simulink model "Hybrid_PV_Wind_System"  (R2018a)
settings: Solver=ode3  StartTime=0.0  StopTime=80  FixedStep=1e-4  RelTol=1e-3  EnableMultiTasking=on
InitFcn:
  | clear all ;
  | clc;
  | 
  | %%Wind System%%
  | 
  | %wind speed
  | Z_data=10;
  | Z_hub=85;
  | Z_0=0.03;
  | 
  | %Turbine
  | R_=45;
  | G=100;
  | lambda_opt=7.07;
  | Rho=1.225;
  | J=254;
  | f=0.01;
  | 
  | %RL filter;
  | 
  | fs=10000;
  | fe=50;
  | Ws=2*pi*fe;
  | Pres=3e6;
  | L=0.75e-3;
  | R=0.075;
  | c=38e-3;
  | 
  | %Commande CCR;
  | 
  | Id_=0;
  | Vdc_=1200;
  | %Vq_=0;
  | tr=0.001;
  | kp=3*L/tr;
  | ki=3*R/tr;
  | 
  | %CCM Commande;
  | 
  | p=2;
  | Tr=0.02;
  | Lfs=121e-6;
  | Lfr=57.3e-6;
  | Lm=12.12e-3;
  | m=1;
  | Ls=Lfs+Lm;
  | Lr=Lfr+m*Lm;
  | sigma=1-(m*Lm)^2/(Ls*Lr);
  | Rr=3.82e-3;
  | Rs=2.97e-3;
  | kpr=3*sigma*Lr/Tr;
  | kir=3*Rr/Tr;
  | Qs_ref=0;
  | 
  | %%PV SYSTEM%%
  | 
  | % T_cellule;
  | NOCT=45;
  | 
  | %PV module;
  | ... (+42 lines)
undefined symbols (not defined in the file): sigbuilder_block
libraries: powerlib_meascontrol x20, simulink x10
(part 2 of 2)

== system Hybrid_PV_Wind_System/August/Temperature8 ==
  Demux : Demux  Tag=STV Demux  Outputs=1
      settings: DisplayOption=none
  FromWs : FromWorkspace  Tag=STV FromWs  VariableName=tuvar
      SigBuilderData=|
      | common.afterFinalStr = 'Extrapolate'
      | common.sampleTime = 0
      | dataSet.timeRange = [0 745]
      | dataSet.name = 'Group 1'
      | sbobj.Groups.Name = 'Group 1'
      | sbobj.Groups.Signals.Name = 'Signal 1'
      | sbobj.Groups.Signals.XData = [0 1 2 3 4 5 6 7 8 9 10 11 ... (745 elements, 1x745)]
      | sbobj.Groups.Signals.YData = [35.7 34 32.3 31.4 30.5 29.9 29.9 31.6 33.8 36 38.1 40 ... (745 elements, 1x745)]
      | sbobj.Groups.TimeRange = [0 745]
  Signal 1 : Outport  Tag=STV Outport
  wires:
  FromWs/1 -> Demux/1
  Demux/1 -> Signal 1/1

== system Hybrid_PV_Wind_System/August/Three Phase DC AC inverter ==
  Vdc : Inport
  pwma : Inport  Port=2
  pwmb : Inport  Port=3
  pwmc : Inport  Port=4
  Fcn : Fcn  Expr=u(1)/6*(2*u(2)-u(3)-u(4))
  Fcn1 : Fcn  Expr=u(1)/6*(-u(2)+2*u(3)-u(4))
  Fcn2 : Fcn  Expr=u(1)/6*(-u(2)-u(3)+2*u(4))
  Mux : Mux
  Via : Outport
  Vib : Outport  Port=2
  Vic : Outport  Port=3
  wires:
  Vdc/1 -> Mux/1
  Mux/1 -> Fcn2/1, Fcn1/1, Fcn/1
  Fcn2/1 -> Vic/1
  Fcn1/1 -> Vib/1
  Fcn/1 -> Via/1
  pwma/1 -> Mux/2
  pwmb/1 -> Mux/3
  pwmc/1 -> Mux/4

== system Hybrid_PV_Wind_System/August/Turbine ==
  note: T_aero
  note: omega_t
  note: omega
  note: lambda
  note: Cp
  S : Inport
  B : Inport  Port=2
  1/lambda_i : Fcn  Expr=1/(u(1)+0.08*u(2))-0.035/(2^3+1)
  Cp(lambda,B) : Fcn  Expr=0.5176*(116*u(2)-0.4*u(3)-5)*exp(-21*u(2))+0.0068*u(1)
  Gain : Gain  Gain=R_/G
  Gain1 : Gain  Gain=1/G
  Gain2 : Gain  Gain=1/G
  Gain3 : Gain  Gain=lambda_opt*G/R_
  Gain5 : Gain  Gain=-1
  Mux : Mux  Inputs=2
  Mux1 : Mux  Inputs=3
  Mux2 : Mux  Inputs=3
  Mux3 : Mux  Inputs=2
  Product : Product  Inputs=*/
  Saturation : Saturate  UpperLimit=200  LowerLimit=0
  Saturation1 : Saturate  UpperLimit=0  LowerLimit=-3e6
  Saturation2 : Saturate  UpperLimit=200  LowerLimit=0
  Scope{1..5} (5 alike) : Scope
  Subsystem : Subsystem
  Subsystem1 : Subsystem
  Subsystem8 : Subsystem
  Taero(S,cp) : Fcn  Expr=0.5*u(1)*Rho*pi*(R_^2)*(u(2)^3)/u(3)
  omega : Outport
  Ps* : Outport  Port=2
  wires:
  Subsystem8/1(Ps*) -> Saturation1/1
  1/lambda_i/1 -> Mux1/2
  B/1 -> Mux1/3, Mux3/2
  Product/1 -> Mux3/1, Mux1/1
  S/1 -> Gain3/1, Mux2/2, Product/2
  Cp(lambda,B)/1 -> Mux2/1
  Gain/1 -> Product/1
  Gain2/1 -> Mux2/3
  Mux1/1 -> Cp(lambda,B)/1
  Mux2/1 -> Taero(S,cp)/1
  Taero(S,cp)/1 -> Gain1/1
  Mux/1 -> Scope1/1
  Mux3/1 -> 1/lambda_i/1
  Gain5/1 -> Subsystem8/1(Tem*), Scope3/1
  Subsystem1/1(Tem) -> Subsystem/2(Tem), Gain5/1
  Gain1/1 -> Scope5/1, Subsystem1/1(Tt), Subsystem/1(Tt)
  Gain3/1 -> Saturation/1, Mux/1
  Saturation/1 -> Subsystem1/2(omega_ref)
  Saturation1/1 -> Scope4/1, Ps*/1
  Subsystem/1(omega) -> Saturation2/1
  Saturation2/1 -> omega/1, Scope2/1, Gain/1, Gain2/1, Mux/2, Subsystem1/3(omega), Subsystem8/2(omega)

== system Hybrid_PV_Wind_System/August/Wind speed8 ==
  Demux : Demux  Tag=STV Demux  Outputs=1
      settings: DisplayOption=none
  FromWs : FromWorkspace  Tag=STV FromWs  VariableName=tuvar
      SigBuilderData=|
      | common.afterFinalStr = 'Extrapolate'
      | common.sampleTime = 0
      | dataSet.timeRange = [0 750]
      | dataSet.name = 'Group 1'
      | sbobj.Groups.Name = 'Group 1'
      | sbobj.Groups.Signals.Name = 'Signal 2'
      | sbobj.Groups.Signals.XData = [0 1 2 3 4 5 6 7 8 9 10 11 ... (744 elements, 1x744)]
      | sbobj.Groups.Signals.YData = [7.2 6.9 7.1 7.1 4.6 5.7 4.8 5.2 4.4 6.2 7.7 8.7 ... (744 elements, 1x744)]
      | sbobj.Groups.TimeRange = [0 750]
  Signal 2 : Outport  Tag=STV Outport
  wires:
  Demux/1 -> Signal 2/1
  FromWs/1 -> Demux/1

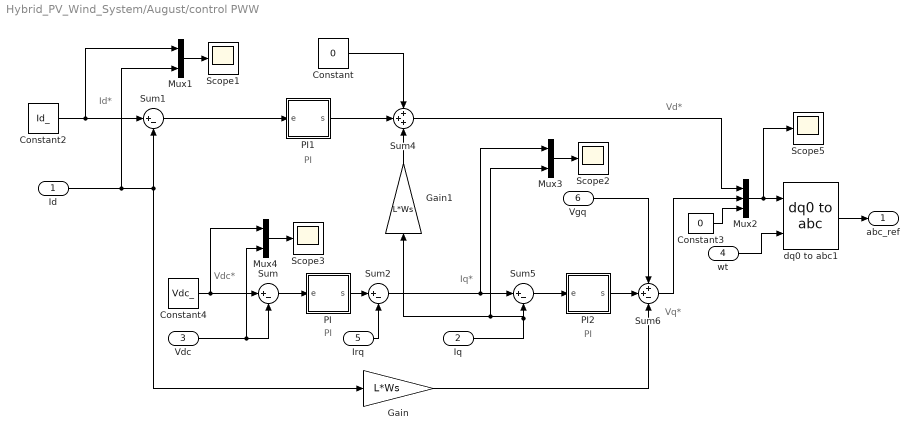
== system Hybrid_PV_Wind_System/August/control PWW  ==
  note: PI
  note: Iq*
  note: Vq*
  note: Vd*
  note: Id*
  note: Vdc*
  note: PI
  note: PI
  Id : Inport
  Iq : Inport  Port=2
  Vdc : Inport  Port=3
  wt : Inport  Port=4
  Irq : Inport  Port=5
  Vgq : Inport  Port=6
  Constant : Constant  Value=0
  Constant2 : Constant  Value=Id_
  Constant3 : Constant  Value=0
  Constant4 : Constant  Value=Vdc_
  Gain : Gain  Gain=L*Ws
  Gain1 : Gain  Gain=L*Ws
  Mux1 : Mux  Inputs=2
  Mux2 : Mux  Inputs=3
  Mux3 : Mux  Inputs=2
  Mux4 : Mux  Inputs=2
  PI : Subsystem
  PI1 : Subsystem
  PI2 : Subsystem
  Scope{1..3,5} (4 alike) : Scope
  Sum{,1..2,5} (4 alike) : Sum  Inputs=|+-
  Sum4 : Sum  Inputs=+++
  Sum6 : Sum  Inputs=++-
  dq0 to abc1 : powerlib_meascontrol/Transformations/dq0 to abc  Alignment=90 degrees behind phase A axis
  abc_ref : Outport
  wires:
  Sum1/1 -> PI1/1(e)
  Sum/1 -> PI/1(e)
  PI/1(s) -> Sum2/1
  Constant2/1 -> Mux1/1, Sum1/1
  PI1/1(s) -> Sum4/2
  Constant3/1 -> Mux2/3
  Mux2/1 -> dq0 to abc1/1, Scope5/1
  dq0 to abc1/1 -> abc_ref/1
  wt/1 -> dq0 to abc1/2
  PI2/1(s) -> Sum6/2
  Id/1 -> Mux1/2, Sum1/2, Gain/1
  Sum6/1 -> Mux2/2
  Sum5/1 -> PI2/1(e)
  Sum4/1 -> Mux2/1
  Vgq/1 -> Sum6/1
  Gain/1 -> Sum6/3
  Irq/1 -> Sum2/2
  Constant/1 -> Sum4/1
  Gain1/1 -> Sum4/3
  Mux1/1 -> Scope1/1
  Sum2/1 -> Sum5/1, Mux3/1
  Iq/1 -> Sum5/2, Mux3/2, Gain1/1
  Mux3/1 -> Scope2/1
  Constant4/1 -> Mux4/1, Sum/1
  Vdc/1 -> Mux4/2, Sum/2
  Mux4/1 -> Scope3/1

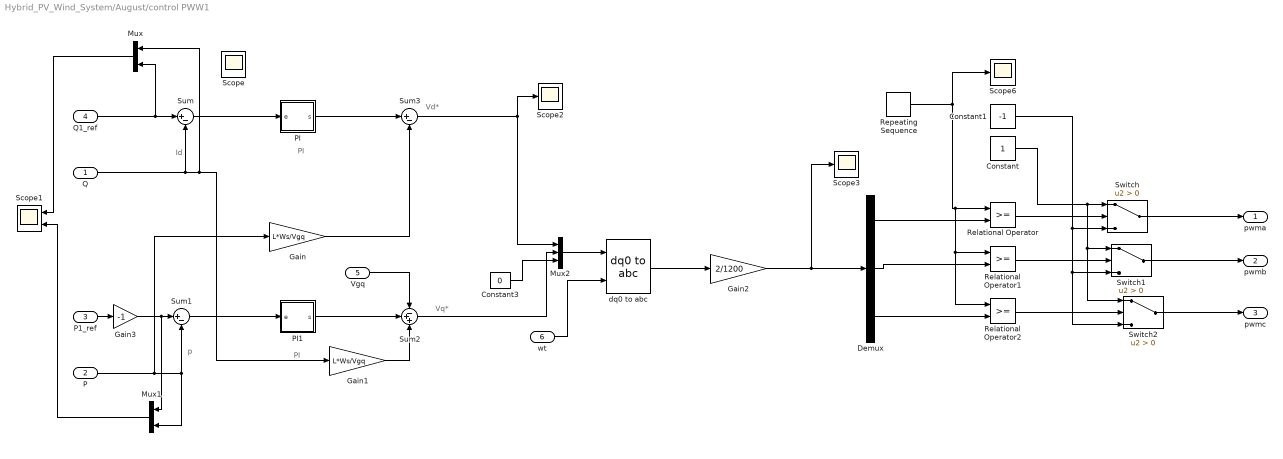
== system Hybrid_PV_Wind_System/August/control PWW1 ==
  note: PI
  note: PI
  note: Vd*
  note: Vq*
  note: p
  note: Id
  "Q " : Inport
  P : Inport  Port=2
  P1_ref : Inport  Port=3
  Q1_ref : Inport  Port=4
  Vgq : Inport  Port=5
  wt : Inport  Port=6
  Constant : Constant
  Constant1 : Constant  Value=-1
  Constant3 : Constant  Value=0
  Demux : Demux  Outputs=3
  Gain : Gain  Gain=L*Ws/Vgq
  Gain1 : Gain  Gain=L*Ws/Vgq
  Gain2 : Gain  Gain=2/1200
  Gain3 : Gain  Gain=-1
  Mux : Mux  Inputs=2
  Mux1 : Mux  Inputs=2
  Mux2 : Mux  Inputs=3
  PI : Subsystem
  PI1 : Subsystem
  Relational Operator : RelationalOperator  OutDataTypeStr=boolean  RndMeth=Nearest
  Relational Operator1 : RelationalOperator  OutDataTypeStr=boolean  RndMeth=Nearest
  Relational Operator2 : RelationalOperator  OutDataTypeStr=boolean  RndMeth=Nearest
  Repeating Sequence : simulink/Sources/Repeating Sequence  rep_seq_t=[0 1/40000 1/20000 3/40000 1/10000]  rep_seq_y="[0 1  0 -1 0]"
  Scope{,2..3,6} (4 alike) : Scope
  Scope1 : Scope  NumInputPorts=2
  Sum : Sum  Inputs=|+-
  Sum1 : Sum  Inputs=|+-
  Sum2 : Sum  Inputs=-++
  Sum3 : Sum  Inputs=|+-
  Switch : Switch  Criteria=u2 > Threshold
  Switch1 : Switch  Criteria=u2 > Threshold
  Switch2 : Switch  Criteria=u2 > Threshold
  dq0 to abc : powerlib_meascontrol/Transformations/dq0 to abc  Alignment=90 degrees behind phase A axis
  pwma : Outport
  pwmb : Outport  Port=2
  pwmc : Outport  Port=3
  wires:
  Sum1/1 -> PI1/1(e)
  "Q "/1 -> Mux/1, Gain1/1, Sum/2
  Sum/1 -> PI/1(e)
  PI/1(s) -> Sum3/1
  P1_ref/1 -> Gain3/1
  Mux/1 -> Scope1/1
  P/1 -> Mux1/2, Sum1/2, Gain/1
  Mux1/1 -> Scope1/2
  PI1/1(s) -> Sum2/2
  Constant3/1 -> Mux2/3
  Q1_ref/1 -> Mux/2, Sum/1
  Repeating Sequence/1 -> Scope6/1, Relational Operator2/1, Relational Operator1/1, Relational Operator/1
  Demux/1 -> Relational Operator/2
  Demux/2 -> Relational Operator1/2
  Demux/3 -> Relational Operator2/2
  Switch2/1 -> pwmc/1
  Switch1/1 -> pwmb/1
  Switch/1 -> pwma/1
  Relational Operator/1 -> Switch/2
  Constant/1 -> Switch1/1, Switch2/1, Switch/1
  Constant1/1 -> Switch/3, Switch1/3, Switch2/3
  Relational Operator1/1 -> Switch1/2
  Relational Operator2/1 -> Switch2/2
  Mux2/1 -> dq0 to abc/1
  Sum3/1 -> Scope2/1, Mux2/1
  Sum2/1 -> Mux2/2
  wt/1 -> dq0 to abc/2
  Vgq/1 -> Sum2/1
  Gain/1 -> Sum3/2
  Gain1/1 -> Sum2/3
  dq0 to abc/1 -> Gain2/1
  Gain2/1 -> Scope3/1, Demux/1
  Gain3/1 -> Mux1/1, Sum1/1

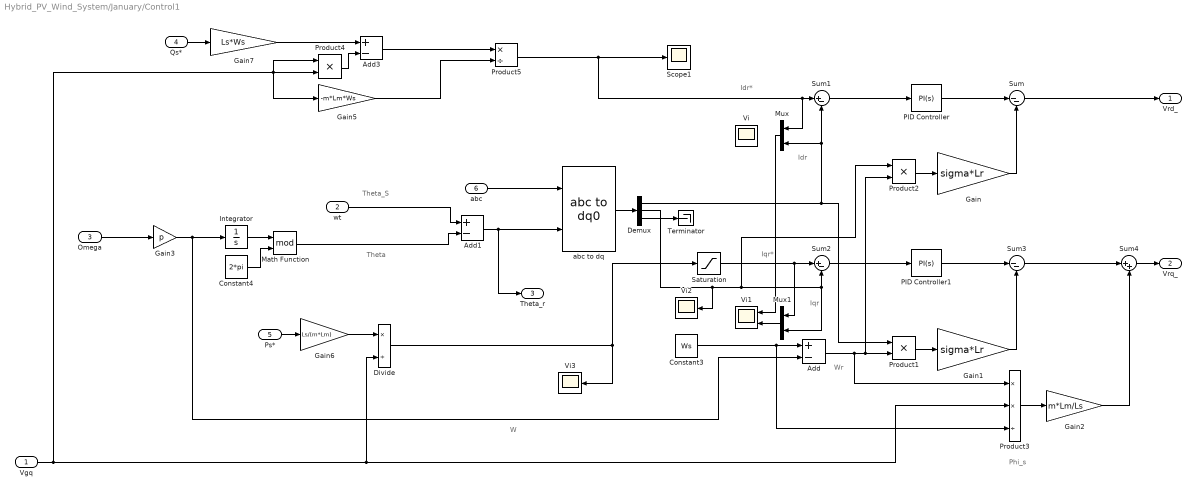
== system Hybrid_PV_Wind_System/January/Control1 ==
  note: Theta_S
  note: Theta
  note: W
  note: Wr
  note: Iqr
  note: Idr
  note: Phi_s
  note: Idr*
  note: Iqr*
  Vgq : Inport
  wt : Inport  Port=2
  Omega : Inport  Port=3
  Qs* : Inport  Port=4
  Ps* : Inport  Port=5
  abc : Inport  Port=6
  Add : Sum  Inputs=+-
  Add1 : Sum  Inputs=+-
  Add3 : Sum  Inputs=+-
  Constant3 : Constant  Value=Ws
  Constant4 : Constant  Value=2*pi
  Demux : Demux  Outputs=3
  Divide : Product  Inputs=*/
  Gain : Gain  Gain=sigma*Lr
  Gain1 : Gain  Gain=sigma*Lr
  Gain2 : Gain  Gain=m*Lm/Ls
  Gain3 : Gain  Gain=p
  Gain5 : Gain  Gain=-m*Lm*Ws
  Gain6 : Gain  Gain=Ls/(m*Lm)
  Gain7 : Gain  Gain=Ls*Ws
  Integrator : Integrator
  Math Function : Math  Operator=mod  SaturateOnIntegerOverflow=on
  Mux : Mux  Inputs=2
  Mux1 : Mux  Inputs=2
  PID Controller : simulink/Continuous/PID Controller  Controller=PI  Form=Parallel  TimeDomain=Continuous-time  SampleTime=-1  IntegratorMethod=Forward Euler  ControllerParametersSource=internal  P=kpr*62  I=kir*62  D=0  N=100  UseFilter=on  TunerSelectOption=Transfer Function Based (PID Tuner App)  InitialConditionSource=internal  InitialConditionForIntegrator=0  InitialConditionForFilter=0  DifferentiatorICPrevScaledInput=0  ExternalReset=none  TrackingMode=off  Kt=1  LimitOutput=off  UpperSaturationLimit=inf  LowerSaturationLimit=-inf  LinearizeAsGain=on  AntiWindupMode=none  Kb=1  POutMin=[]  POutMax=[]  IOutMin=[]  IOutMax=[]  DOutMin=[]  DOutMax=[]  NOutMin=[]  NOutMax=[]  SumOutMin=[]  SumOutMax=[]  SaturationOutMin=[]  SaturationOutMax=[]  PParamMin=[]  PParamMax=[]  IParamMin=[]  IParamMax=[]  DParamMin=[]  DParamMax=[]  NParamMin=[]  NParamMax=[]  KbParamMin=[]  KbParamMax=[]  KtParamMin=[]  KtParamMax=[]  KbOutMin=[]  KbOutMax=[]  KtOutMin=[]  KtOutMax=[]  IntegratorOutMin=[]  IntegratorOutMax=[]  FilterOutMin=[]  FilterOutMax=[]  SumI1OutMin=[]  SumI1OutMax=[]  SumI2OutMin=[]  SumI2OutMax=[]  SumI3OutMin=[]  SumI3OutMax=[]  SumDOutMin=[]  SumDOutMax=[]  DifferentiatorOutMin=[]  DifferentiatorOutMax=[]  FilterDiffOutCoefMin=[]  FilterDiffOutCoefMax=[]  ReciprocalOutMin=[]  ReciprocalOutMax=[]  SumDenOutMin=[]  SumDenOutMax=[]  SumNumOutMin=[]  SumNumOutMax=[]  DivideOutMin=[]  DivideOutMax=[]  IntegratorContinuousStateAttributes=''  IntegratorStateMustResolveToSignalObject=off  IntegratorRTWStateStorageClass=Auto  FilterContinuousStateAttributes=''  FilterStateMustResolveToSignalObject=off  FilterRTWStateStorageClass=Auto
  PID Controller1 : simulink/Continuous/PID Controller  Controller=PI  Form=Parallel  TimeDomain=Continuous-time  SampleTime=-1  IntegratorMethod=Forward Euler  ControllerParametersSource=internal  P=kpr*62  I=kir*62  D=0  N=100  UseFilter=on  TunerSelectOption=Transfer Function Based (PID Tuner App)  InitialConditionSource=internal  InitialConditionForIntegrator=0  InitialConditionForFilter=0  DifferentiatorICPrevScaledInput=0  ExternalReset=none  TrackingMode=off  Kt=1  LimitOutput=off  UpperSaturationLimit=inf  LowerSaturationLimit=-inf  LinearizeAsGain=on  AntiWindupMode=none  Kb=1  POutMin=[]  POutMax=[]  IOutMin=[]  IOutMax=[]  DOutMin=[]  DOutMax=[]  NOutMin=[]  NOutMax=[]  SumOutMin=[]  SumOutMax=[]  SaturationOutMin=[]  SaturationOutMax=[]  PParamMin=[]  PParamMax=[]  IParamMin=[]  IParamMax=[]  DParamMin=[]  DParamMax=[]  NParamMin=[]  NParamMax=[]  KbParamMin=[]  KbParamMax=[]  KtParamMin=[]  KtParamMax=[]  KbOutMin=[]  KbOutMax=[]  KtOutMin=[]  KtOutMax=[]  IntegratorOutMin=[]  IntegratorOutMax=[]  FilterOutMin=[]  FilterOutMax=[]  SumI1OutMin=[]  SumI1OutMax=[]  SumI2OutMin=[]  SumI2OutMax=[]  SumI3OutMin=[]  SumI3OutMax=[]  SumDOutMin=[]  SumDOutMax=[]  DifferentiatorOutMin=[]  DifferentiatorOutMax=[]  FilterDiffOutCoefMin=[]  FilterDiffOutCoefMax=[]  ReciprocalOutMin=[]  ReciprocalOutMax=[]  SumDenOutMin=[]  SumDenOutMax=[]  SumNumOutMin=[]  SumNumOutMax=[]  DivideOutMin=[]  DivideOutMax=[]  IntegratorContinuousStateAttributes=''  IntegratorStateMustResolveToSignalObject=off  IntegratorRTWStateStorageClass=Auto  FilterContinuousStateAttributes=''  FilterStateMustResolveToSignalObject=off  FilterRTWStateStorageClass=Auto
  Product1 : Product
  Product2 : Product
  Product3 : Product  Inputs=**/
  Product4 : Product  Inputs=**
  Product5 : Product  Inputs=*/
  Saturation : Saturate  UpperLimit=8e3  LowerLimit=-8e3
  Scope1 : Scope
  Sum : Sum  Inputs=|--
  Sum1 : Sum  Inputs=|+-
  Sum2 : Sum  Inputs=|+-
  Sum3 : Sum  Inputs=|--
  Sum4 : Sum  Inputs=|++
  Terminator : Terminator
  Vi : Scope
  Vi1 : Scope  NumInputPorts=2
  Vi2 : Scope
  Vi3 : Scope
  abc to dq : powerlib_meascontrol/Transformations/abc to dq0  Alignment=90 degrees behind phase A axis
  Vrd_ : Outport
  Vrq_ : Outport  Port=2
  Theta_r : Outport  Port=3
  wires:
  Sum2/1 -> PID Controller1/1
  Sum1/1 -> PID Controller/1
  Demux/2 -> Vi2/1, Mux1/2, Sum2/2, Product2/1
  PID Controller/1 -> Sum/1
  Gain/1 -> Sum/2
  Sum4/1 -> Vrq_/1
  PID Controller1/1 -> Sum3/1
  Demux/1 -> Sum1/2, Mux/2, Product1/1
  Gain2/1 -> Sum4/2
  Sum3/1 -> Sum4/1
  Sum/1 -> Vrd_/1
  Gain1/1 -> Sum3/2
  Constant3/1 -> Product3/3, Add/1
  Product1/1 -> Gain1/1
  Add/1 -> Product3/1, Product2/2, Product1/2
  Omega/1 -> Gain3/1
  Product2/1 -> Gain/1
  Product3/1 -> Gain2/1
  abc to dq/1 -> Demux/1
  Demux/3 -> Terminator/1
  abc/1 -> abc to dq/1
  wt/1 -> Add1/1
  Integrator/1 -> Math Function/1
  Constant4/1 -> Math Function/2
  Math Function/1 -> Add1/2
  Gain3/1 -> Integrator/1, Add/2
  Mux/1 -> Vi1/1
  Mux1/1 -> Vi1/2
  Add1/1 -> abc to dq/2, Theta_r/1
  Add3/1 -> Product5/1
  Vgq/1 -> Product3/2, Divide/2, Product4/1, Gain5/1, Product4/2
  Qs*/1 -> Gain7/1
  Gain5/1 -> Product5/2
  Product5/1 -> Sum1/1, Mux/1, Scope1/1
  Ps*/1 -> Gain6/1
  Gain6/1 -> Divide/1
  Gain7/1 -> Add3/1
  Product4/1 -> Add3/2
  Divide/1 -> Vi3/1, Saturation/1
  Saturation/1 -> Mux1/1, Sum2/1

== system Hybrid_PV_Wind_System/January/DC//DC boost ==
  Vpv : Inport
  Ipv : Inport  Port=2
  Add : Sum  Inputs=+-
  Gain : Gain  Gain=1/l
  Gain1 : Gain  Gain=1/l
  Gain2 : Gain  Gain=1/C
  Gain3 : Gain  Gain=1/(r*C)
  Integrator : Integrator
  Integrator1 : Integrator
  Product : Product
  Product1 : Product
  Product2 : Product  Inputs=*/
  Product4 : Product
  Sum : Sum  Inputs=|+-
  Sum1 : Sum  Inputs=|+-
  Sum2 : Sum  Inputs=|+-
  const : Constant
  const2 : Constant  Value=Vdc
  iL : Outport
  Is : Outport  Port=2
  Vdc : Outport  Port=3
  wires:
  Gain3/1 -> Sum2/2
  Integrator1/1 -> Vdc/1, Product/2, Gain3/1
  Sum2/1 -> Integrator1/1
  Product1/1 -> Gain2/1
  Product/1 -> Gain1/1
  Sum1/1 -> Integrator/1
  Gain1/1 -> Sum1/2
  Gain2/1 -> Sum2/1
  Gain/1 -> Sum1/1
  Add/1 -> Sum/2
  const/1 -> Add/1, Sum/1
  Vpv/1 -> Product2/1, Gain/1
  const2/1 -> Product2/2
  Product2/1 -> Add/2
  Sum/1 -> Product/1, Product4/1, Product1/1
  Integrator/1 -> iL/1, Product1/2
  Product4/1 -> Is/1
  Ipv/1 -> Product4/2

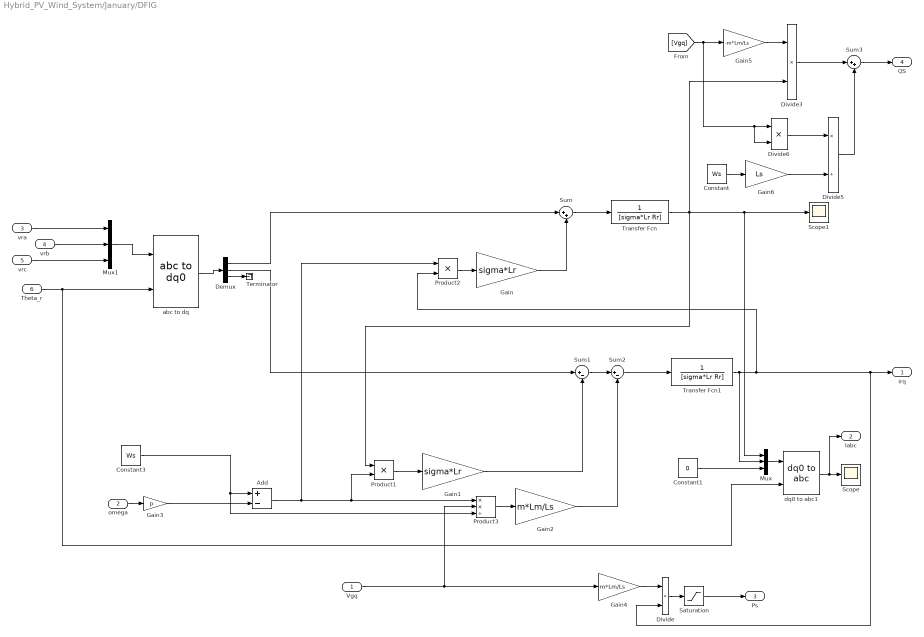
== system Hybrid_PV_Wind_System/January/DFIG  ==
  Vgq : Inport
  omega : Inport  Port=2
  vra : Inport  Port=3
  vrb : Inport  Port=4
  vrc : Inport  Port=5
  Theta_r : Inport  Port=6
  Add : Sum  Inputs=+-
  Constant : Constant  Value=Ws
  Constant1 : Constant  Value=0
  Constant3 : Constant  Value=Ws
  Demux : Demux  Outputs=3
  Divide : Product  Inputs=**
  Divide3 : Product  Inputs=**
  Divide5 : Product  Inputs=*/
  Divide6 : Product  Inputs=**
  Gain : Gain  Gain=sigma*Lr
  Gain1 : Gain  Gain=sigma*Lr
  Gain2 : Gain  Gain=m*Lm/Ls
  Gain3 : Gain  Gain=p
  Gain4 : Gain  Gain=m*Lm/Ls
  Gain5 : Gain  Gain=-m*Lm/Ls
  Gain6 : Gain  Gain=Ls
  Mux : Mux  Inputs=3
  Mux1 : Mux  Inputs=3
  Product1 : Product
  Product2 : Product
  Product3 : Product  Inputs=**/
  Saturation : Saturate  UpperLimit=0  LowerLimit=-3e6
  Scope : Scope
  Scope1 : Scope
  Sum : Sum  Inputs=|++
  Sum1 : Sum  Inputs=|+-
  Sum2 : Sum  Inputs=|+-
  Sum3 : Sum  Inputs=|++
  Terminator : Terminator
  Transfer Fcn : TransferFcn  Denominator=[sigma*Lr Rr]
  Transfer Fcn1 : TransferFcn  Denominator=[sigma*Lr Rr]
  abc to dq : powerlib_meascontrol/Transformations/abc to dq0  Alignment=90 degrees behind phase A axis
  dq0 to abc1 : powerlib_meascontrol/Transformations/dq0 to abc  Alignment=90 degrees behind phase A axis
  irq : Outport
  Iabc : Outport  Port=2
  Ps : Outport  Port=3
  QS : Outport  Port=4
  wires:
  Transfer Fcn/1 -> Scope1/1, Mux/1, Divide3/2, Product1/1
  Sum/1 -> Transfer Fcn/1
  Demux/2 -> Sum1/1
  Demux/1 -> Sum/1
  Product2/1 -> Gain/1
  Gain/1 -> Sum/2
  Constant3/1 -> Product3/3, Add/1
  Product1/1 -> Gain1/1
  Product3/1 -> Gain2/1
  Sum1/1 -> Sum2/1
  Gain1/1 -> Sum1/2
  Gain2/1 -> Sum2/2
  Sum2/1 -> Transfer Fcn1/1
  Add/1 -> Product2/1, Product1/2, Product3/1
  omega/1 -> Gain3/1
  Gain3/1 -> Add/2
  Constant1/1 -> Mux/3
  Mux/1 -> dq0 to abc1/1
  dq0 to abc1/1 -> Iabc/1, Scope/1
  abc to dq/1 -> Demux/1
  Demux/3 -> Terminator/1
  Mux1/1 -> abc to dq/1
  vra/1 -> Mux1/1
  vrb/1 -> Mux1/2
  vrc/1 -> Mux1/3
  Theta_r/1 -> dq0 to abc1/2, abc to dq/2
  Transfer Fcn1/1 -> irq/1, Divide/2, Product2/2, Mux/2
  Divide/1 -> Saturation/1
  Gain4/1 -> Divide/1
  Gain5/1 -> Divide3/1
  Divide3/1 -> Sum3/1
  Sum3/1 -> QS/1
  [Vgq] -> Divide6/2, Divide6/1, Gain5/1
  Divide6/1 -> Divide5/1
  Gain6/1 -> Divide5/2
  Constant/1 -> Gain6/1
  Divide5/1 -> Sum3/2
  Vgq/1 -> Product3/2, Gain4/1
  Saturation/1 -> Ps/1

== system Hybrid_PV_Wind_System/January/DHI ==
  Demux : Demux  Tag=STV Demux  Outputs=1
      settings: DisplayOption=none
  FromWs : FromWorkspace  Tag=STV FromWs  VariableName=tuvar
      SigBuilderData=|
      | common.afterFinalStr = 'Extrapolate'
      | common.sampleTime = 0
      | dataSet.timeRange = [0 750]
      | dataSet.name = 'Group 1'
      | sbobj.Groups.Name = 'Group 1'
      | sbobj.Groups.Signals.Name = 'Signal 1'
      | sbobj.Groups.Signals.XData = [0 1 2 3 4 5 6 7 8 9 10 11 ... (744 elements, 1x744)]
      | sbobj.Groups.Signals.YData = [0 0 0 0 0 0 0 0 40 51 53 60 67 68 62 54 52 37 0 0 0 0 0 0 0 0 0 0 0 0 0 0 33 46 51 59 65 66 60 51 47 37 0 0 0 0 0 0 0 0 0 0 0 0 0 0 33 46 50 60 67 68 64 55 50 32 0 0 0 0 0 0 0 0 0 0 0 0 0 0 33 46 51 62 69 71 66 58 53 32 1 0 0 0 0 0 0 0 0 0 0 0 0 0 40 51 53 60 67 68 63 55 52 39 0 0 0 0 0 0 0 0 0 0 0 0 0 0 33 46 51 59 66 67 61 52 47 35 1 0 0 0 0 0 0 0 0 0 0 0 0 0 33 51 51 60 66 67 61 52 47 37 1 0 0 0 0 0 0 0 0 0 0 0 0 0 33 50 51 60 67 68 62 53 48 39 0 0 0 0 0 0 0 0 0 0 0 0 0 0 33 46 51 61 68 68 64 56 50 33 1 0 0 0 0 0 0 0 0 0 0 0 0 0 33 46 51 60 66 67 62 52 48 36 1 0 0 0 0 0 0 0 0 0 0 0 0 0 34 50 51 60 67 68 62 53 48 38 1 0 0 0 0 0 0 0 0 0 0 0 0 0 40 51 53 62 68 70 63 54 49 39 1 0 0 0 0 0 0 0 0 0 0 0 0 0 40 52 54 64 69 70 65 56 50 40 1 0 0 0 0 0 0 0 0 0 0 0 0 0 40 51 53 62 68 68 63 53 48 36 2 0 0 0 0 0 0 0 0 0 0 0 0 0 33 46 51 61 69 69 63 53 48 38 1 0 0 0 0 0 0 0 0 0 0 0 0 0 33 46 51 61 68 70 65 56 49 36 2 0 0 0 0 0 0 0 0 0 0 0 0 0 33 46 51 62 70 72 66 57 51 37 2 0 0 0 0 0 0 0 0 0 0 0 0 0 34 46 51 61 69 71 67 57 51 37 3 0 0 0 0 0 0 0 0 0 0 0 0 0 35 51 52 62 69 70 64 54 48 38 3 0 0 0 0 0 0 0 0 0 0 0 0 0 41 51 55 64 71 72 65 55 49 40 3 0 0 0 0 0 0 0 0 0 0 0 0 0 41 52 54 64 72 74 69 58 58 45 2 0 0 0 0 0 0 0 0 0 0 0 0 0 41 52 55 66 73 74 68 59 52 38 3 0 0 0 0 0 0 0 0 0 0 0 0 0 32 49 55 66 74 75 70 60 53 35 3 0 0 0 0 0 0 0 0 0 0 0 0 0 33 47 53 63 71 72 66 56 49 32 3 0 0 0 0 0 0 0 0 0 0 0 0 0 35 47 53 64 73 76 69 58 51 41 4 0 0 0 0 0 0 0 0 0 0 0 0 0 42 52 57 68 77 78 71 58 51 32 4 0 0 0 0 0 0 0 0 0 0 0 0 0 37 56 60 71 79 78 72 63 56 32 5 0 0 0 0 0 0 0 0 0 0 0 0 0 37 51 56 66 75 76 70 60 52 24 6 0 0 0 0 0 0 0 0 0 0 0 0 0 38 55 62 72 79 83 81 71 64 43 5 0 0 0 0 0 0 0 0 0 0 0 0 0 39 60 67 80 87 83 74 61 54 36 8 0 0 0 0 0 0 0 0 0 0 0 0 0 39 58 74 74 82 91 79 63 56 36 7 0 0 0 0 0]
      | sbobj.Groups.TimeRange = [0 750]
  Signal 1 : Outport  Tag=STV Outport
  wires:
  FromWs/1 -> Demux/1
  Demux/1 -> Signal 1/1

== system Hybrid_PV_Wind_System/January/DNI ==
  Demux : Demux  Tag=STV Demux  Outputs=1
      settings: DisplayOption=none
  FromWs : FromWorkspace  Tag=STV FromWs  VariableName=tuvar
      SigBuilderData=|
      | common.afterFinalStr = 'Extrapolate'
      | common.sampleTime = 0
      | dataSet.timeRange = [0 750]
      | dataSet.name = 'Group 1'
      | sbobj.Groups.Name = 'Group 1'
      | sbobj.Groups.Signals.Name = 'Signal 1'
      | sbobj.Groups.Signals.XData = [0 1 2 3 4 5 6 7 8 9 10 11 ... (744 elements, 1x744)]
      | sbobj.Groups.Signals.YData = [0 0 0 0 0 0 0 0 412 741 884 945 ... (744 elements, 1x744)]
      | sbobj.Groups.TimeRange = [0 750]
  Signal 1 : Outport  Tag=STV Outport
  wires:
  FromWs/1 -> Demux/1
  Demux/1 -> Signal 1/1

== system Hybrid_PV_Wind_System/January/GHI ==
  Demux : Demux  Tag=STV Demux  Outputs=1
      settings: DisplayOption=none
  FromWs : FromWorkspace  Tag=STV FromWs  VariableName=tuvar
      SigBuilderData=|
      | common.afterFinalStr = 'Extrapolate'
      | common.sampleTime = 0
      | dataSet.timeRange = [0 750]
      | dataSet.name = 'Group 1'
      | sbobj.Groups.Name = 'Group 1'
      | sbobj.Groups.Signals.Name = 'Signal 1'
      | sbobj.Groups.Signals.XData = [0 1 2 3 4 5 6 7 8 9 10 11 ... (744 elements, 1x744)]
      | sbobj.Groups.Signals.YData = [0 0 0 0 0 0 0 0 89 276 456 593 ... (744 elements, 1x744)]
      | sbobj.Groups.TimeRange = [0 750]
  Signal 1 : Outport  Tag=STV Outport
  wires:
  Demux/1 -> Signal 1/1
  FromWs/1 -> Demux/1

== system Hybrid_PV_Wind_System/January/Gm1 ==
  Hour : Inport
  DNI : Inport  Port=2
  DHI : Inport  Port=3
  GHI : Inport  Port=4
  Irradiation : MATLAB Function  TreatAsAtomicUnit=on
  G_m : Outport
  wires:
  DHI/1 -> Irradiation/3(o)
  Irradiation/1(y) -> G_m/1
  DNI/1 -> Irradiation/2(k)
  GHI/1 -> Irradiation/4(p)
  Hour/1 -> Irradiation/1(i)

== system Hybrid_PV_Wind_System/January/Grid 1 ==
  Add1 : Sum  Inputs=-+
  Clock : Clock
  Constant : Constant  Value=2*pi
  Constant1 : Constant  Value=pi/2
  Demux : Demux  Outputs=3
  Gain : Gain  Gain=2*pi*50
  Manual Switch : ManualSwitch
  Math Function : Math  Operator=mod  SaturateOnIntegerOverflow=on
  Mux1 : Mux  Inputs=2
  PLL (3ph) : powerlib_meascontrol/PLL/PLL (3ph)  Fmin=45  Par_Init=[0, 50]  ParK=[180, 3200, 1]  TcD=1e-4  MaxRateChangeFreq=12  FilterCutOffFreq=25  Ts=0  AGC=on
  Scope : Scope
  Scope1 : Scope
  Terminator1 : Terminator
  Terminator2 : Terminator
  abc to dq1 : powerlib_meascontrol/Transformations/abc to dq0  Alignment=90 degrees behind phase A axis
  source : Sin  Amplitude=690*sqrt(2)/sqrt(3)  Frequency=2*pi*50  Phase=[0 -2*pi/3 2*pi/3]  SampleTime=0
  Vgd : Outport
  wt : Outport  Port=2
  Vgq : Outport  Port=3
  wires:
  abc to dq1/1 -> Demux/1
  source/1 -> abc to dq1/1, PLL (3ph)/1
  Demux/2 -> Mux1/2, Vgq/1
  Demux/3 -> Terminator1/1
  PLL (3ph)/1 -> Terminator2/1
  Clock/1 -> Gain/1
  PLL (3ph)/2 -> Manual Switch/1
  Gain/1 -> Math Function/1
  Constant/1 -> Math Function/2
  Math Function/1 -> Manual Switch/2
  Add1/1 -> abc to dq1/2, wt/1
  Mux1/1 -> Scope/1
  Constant1/1 -> Add1/1
  Manual Switch/1 -> Add1/2
  Demux/1 -> Mux1/1, Scope1/1, Vgd/1

== system Hybrid_PV_Wind_System/January/Hours ==
  Demux : Demux  Tag=STV Demux  Outputs=1
      settings: DisplayOption=none
  FromWs : FromWorkspace  Tag=STV FromWs  VariableName=tuvar
      SigBuilderData=|
      | common.afterFinalStr = 'Extrapolate'
      | common.sampleTime = 0
      | dataSet.timeRange = [0 750]
      | dataSet.name = 'Group 1'
      | sbobj.Groups.Name = 'Group 1'
      | sbobj.Groups.Signals.Name = 'Signal 1'
      | sbobj.Groups.Signals.XData = [0 1 2 3 4 5 6 7 8 9 10 11 ... (745 elements, 1x745)]
      | sbobj.Groups.Signals.YData = [0 1 2 3 4 5 6 7 8 9 10 11 ... (745 elements, 1x745)]
      | sbobj.Groups.TimeRange = [0 750]
  Signal 1 : Outport  Tag=STV Outport
  wires:
  Demux/1 -> Signal 1/1
  FromWs/1 -> Demux/1

== system Hybrid_PV_Wind_System/January/Hub height spped1 ==
  V : Inport
  Constant : Constant  Value=Z_hub
  Constant5 : Constant  Value=Z_data
  Constant6 : Constant  Value=Z_0
  Divide : Product  Inputs=*/
  Divide1 : Product  Inputs=*/
  Divide2 : Product  Inputs=*/
  Math Function : Math  Operator=log  SaturateOnIntegerOverflow=on
  Math Function1 : Math  Operator=log  SaturateOnIntegerOverflow=on
  Product : Product
  V_hub : Outport
  wires:
  Divide1/1 -> Math Function/1
  Divide2/1 -> Product/1
  Constant6/1 -> Divide1/2, Divide/2
  Constant5/1 -> Divide1/1
  Divide/1 -> Math Function1/1
  Constant/1 -> Divide/1
  Math Function1/1 -> Divide2/1
  Math Function/1 -> Divide2/2
  Product/1 -> V_hub/1
  V/1 -> Product/2

== system Hybrid_PV_Wind_System/January/MPPT1 ==
  I : Inport
  V : Inport  Port=2
  CI : MATLAB Function  TreatAsAtomicUnit=on
  DP : Sum  Inputs=+-
  DV1 : Sum  Inputs=+-
  Memory2 : Memory
  Pk : Product  Inputs=**
  Pk-1 : Memory  InitialCondition=-0.1
  Unit Delay1 : UnitDelay  SampleTime=1e-4  HasFrameUpgradeWarning=on
  Vmpp : Outport
  wires:
  DP/1 -> CI/2(DP)
  DV1/1 -> CI/1(DV)
  CI/1(d) -> Unit Delay1/1
  Pk-1/1 -> DP/2
  Pk/1 -> Pk-1/1, DP/1
  V/1 -> Pk/1, Memory2/1, DV1/1
  Memory2/1 -> DV1/2
  I/1 -> Pk/2
  Unit Delay1/1 -> Vmpp/1

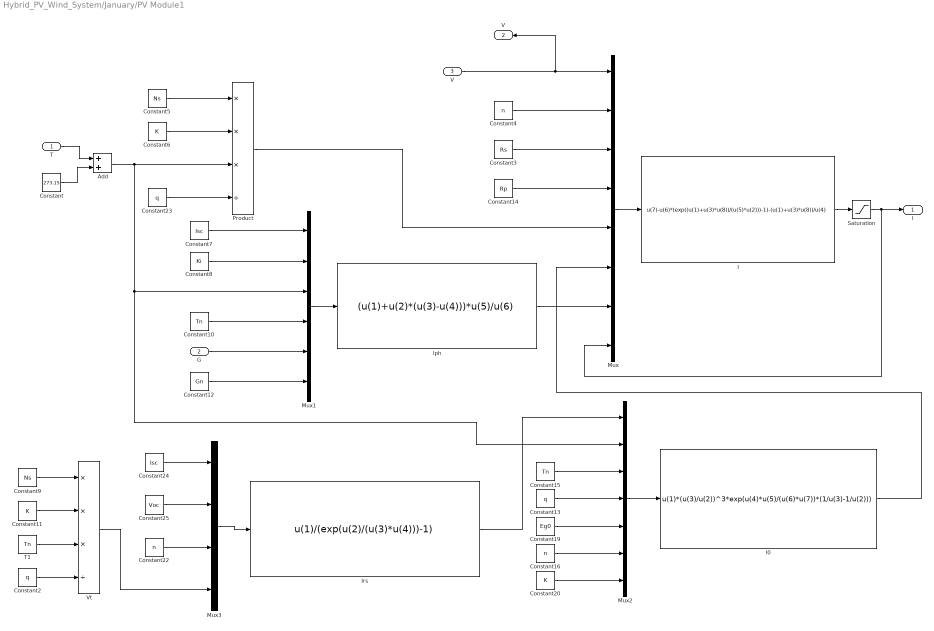
== system Hybrid_PV_Wind_System/January/PV Module1 ==
  T : Inport
  G : Inport  Port=2
  "V " : Inport  Port=3
  Add : Sum
  Constant : Constant  Value=273.15
  Constant10 : Constant  Value=Tn
  Constant11 : Constant  Value=K
  Constant12 : Constant  Value=Gn
  Constant13 : Constant  Value=q
  Constant14 : Constant  Value=Rp
  Constant15 : Constant  Value=Tn
  Constant16 : Constant  Value=n
  Constant19 : Constant  Value=Eg0
  Constant2 : Constant  Value=q
  Constant20 : Constant  Value=K
  Constant22 : Constant  Value=n
  Constant23 : Constant  Value=q
  Constant24 : Constant  Value=Isc
  Constant25 : Constant  Value=Voc
  Constant3 : Constant  Value=Rs
  Constant4 : Constant  Value=n
  Constant5 : Constant  Value=Ns
  Constant6 : Constant  Value=K
  Constant7 : Constant  Value=Isc
  Constant8 : Constant  Value=Ki
  Constant9 : Constant  Value=Ns
  "I " : Fcn  Expr=u(7)-u(6)*(exp((u(1)+u(3)*u(8))/(u(5)*u(2)))-1)-(u(1)+u(3)*u(8))/u(4)
  I0 : Fcn  Expr=u(1)*(u(3)/u(2))^3*exp(u(4)*u(5)/(u(6)*u(7))*(1/u(3)-1/u(2)))
  Iph : Fcn  Expr=(u(1)+u(2)*(u(3)-u(4)))*u(5)/u(6)
  Irs : Fcn  Expr=u(1)/(exp(u(2)/(u(3)*u(4)))-1)
  Mux : Mux  Inputs=8
  Mux1 : Mux  Inputs=6
  Mux2 : Mux  Inputs=7
  Mux3 : Mux
  Product : Product  Inputs=***/
  Saturation : Saturate  UpperLimit=10  LowerLimit=0
  T1 : Constant  Value=Tn
  Vt : Product  Inputs=***/
  I : Outport
  V : Outport  Port=2
  wires:
  Constant5/1 -> Product/1
  Constant20/1 -> Mux2/7
  Constant4/1 -> Mux/2
  Constant3/1 -> Mux/3
  Product/1 -> Mux/5
  "V "/1 -> V/1, Mux/1
  Mux/1 -> "I "/1
  Constant14/1 -> Mux/4
  Mux1/1 -> Iph/1
  Constant8/1 -> Mux1/2
  Constant10/1 -> Mux1/4
  G/1 -> Mux1/5
  Iph/1 -> Mux/7
  Constant7/1 -> Mux1/1
  Constant12/1 -> Mux1/6
  Constant15/1 -> Mux2/3
  Mux2/1 -> I0/1
  Constant13/1 -> Mux2/4
  Constant19/1 -> Mux2/5
  I0/1 -> Mux/6
  Constant16/1 -> Mux2/6
  Add/1 -> Mux2/2, Mux1/3, Product/3
  Mux3/1 -> Irs/1
  Constant24/1 -> Mux3/1
  Constant22/1 -> Mux3/3
  Constant25/1 -> Mux3/2
  Irs/1 -> Mux2/1
  Constant2/1 -> Vt/4
  T1/1 -> Vt/3
  Constant9/1 -> Vt/1
  Constant11/1 -> Vt/2
  Vt/1 -> Mux3/4
  Constant6/1 -> Product/2
  Constant23/1 -> Product/4
  "I "/1 -> Saturation/1
  Constant/1 -> Add/2
  T/1 -> Add/1
  Saturation/1 -> I/1, Mux/8

== system Hybrid_PV_Wind_System/January/PWM ==
  Vrd_ : Inport
  Vrq_ : Inport  Port=2
  theta_r : Inport  Port=3
  Constant : Constant  Value=0
  Constant1 : Constant
  Constant2 : Constant  Value=-1
  Demux1 : Demux  Outputs=3
  Mux2 : Mux  Inputs=3
  Relational Operator : RelationalOperator  OutDataTypeStr=boolean  RndMeth=Nearest
  Relational Operator1 : RelationalOperator  OutDataTypeStr=boolean  RndMeth=Nearest
  Relational Operator2 : RelationalOperator  OutDataTypeStr=boolean  RndMeth=Nearest
  Repeating Sequence : simulink/Sources/Repeating Sequence  rep_seq_t=[0 1/40000 1/20000 3/40000 1/10000]  rep_seq_y="[0 600  0 -600 0]"
  Scope3 : Scope
  Scope5 : Scope
  Scope6 : Scope
  Switch : Switch  Criteria=u2 > Threshold
  Switch1 : Switch  Criteria=u2 > Threshold
  Switch2 : Switch  Criteria=u2 > Threshold
  dq0 to abc1 : powerlib_meascontrol/Transformations/dq0 to abc  Alignment=90 degrees behind phase A axis
  PWMa : Outport
  PWMb : Outport  Port=2
  PWMc : Outport  Port=3
  wires:
  Constant/1 -> Mux2/3
  Switch2/1 -> PWMc/1
  Switch1/1 -> PWMb/1
  Switch/1 -> PWMa/1
  Demux1/2 -> Relational Operator1/2
  Demux1/3 -> Relational Operator2/2
  Demux1/1 -> Relational Operator/2
  Repeating Sequence/1 -> Scope6/1, Relational Operator2/1, Relational Operator1/1, Relational Operator/1
  Constant2/1 -> Switch/3, Switch1/3, Switch2/3
  Mux2/1 -> dq0 to abc1/1, Scope5/1
  Relational Operator2/1 -> Switch2/2
  Vrd_/1 -> Mux2/1
  Constant1/1 -> Switch1/1, Switch2/1, Switch/1
  Relational Operator/1 -> Switch/2
  Relational Operator1/1 -> Switch1/2
  Vrq_/1 -> Mux2/2
  theta_r/1 -> dq0 to abc1/2
  dq0 to abc1/1 -> Demux1/1, Scope3/1

== system Hybrid_PV_Wind_System/January/RL Filtre1 ==
  note: RL filter
  note: DC Bus
  note: Id
  note: Iq
  abc : Inport
  Vgd : Inport  Port=2
  wt : Inport  Port=3
  Vgq : Inport  Port=4
  Irq : Inport  Port=5
  Add : Sum
  Demux1 : Demux  Outputs=3
  Gain : Gain  Gain=L*Ws
  Gain1 : Gain  Gain=1/c
  Gain2 : Gain  Gain=L*Ws
  Integrator : Integrator  UpperSaturationLimit=2000  LowerSaturationLimit=-2000
  Sum : Sum  Inputs=-+-
  Sum2 : Sum  Inputs=-++
  Terminator : Terminator
  Transfer Fcn : TransferFcn  Denominator=[L R]
  Transfer Fcn1 : TransferFcn  Denominator=[L R]
  abc to dq1 : powerlib_meascontrol/Transformations/abc to dq0  Alignment=90 degrees behind phase A axis
  Id : Outport
  Iq : Outport  Port=2
  Vdc : Outport  Port=3
  wires:
  Transfer Fcn1/1 -> Iq/1, Add/1, Gain/1
  abc to dq1/1 -> Demux1/1
  Demux1/3 -> Terminator/1
  abc/1 -> abc to dq1/1
  wt/1 -> abc to dq1/2
  Sum/1 -> Transfer Fcn/1
  Sum2/1 -> Transfer Fcn1/1
  Gain/1 -> Sum/3
  Gain2/1 -> Sum2/3
  Add/1 -> Gain1/1
  Gain1/1 -> Integrator/1
  Transfer Fcn/1 -> Id/1, Gain2/1
  Demux1/2 -> Sum2/2
  Demux1/1 -> Sum/2
  Irq/1 -> Add/2
  Vgq/1 -> Sum2/1
  Vgd/1 -> Sum/1
  Integrator/1 -> Vdc/1

== system Hybrid_PV_Wind_System/January/RL Filtre2 ==
  abc : Inport
  Vgq : Inport  Port=2
  wt : Inport  Port=3
  Demux1 : Demux  Outputs=3
  Gain : Gain  Gain=L*Ws/Vgq
  Gain2 : Gain  Gain=L*Ws/Vgq
  Sum : Sum  Inputs=-++
  Sum1 : Sum  Inputs=|+-
  Terminator : Terminator
  Transfer Fcn : TransferFcn  Denominator="[L1/Vgq  R1/Vgq ]"
  Transfer Fcn1 : TransferFcn  Denominator="[L1/Vgq  R1/Vgq ]"
  abc to dq : powerlib_meascontrol/Transformations/abc to dq0  Alignment=90 degrees behind phase A axis
  "Q " : Outport
  P : Outport  Port=2
  wires:
  Transfer Fcn/1 -> "Q "/1, Gain2/1
  Demux1/1 -> Sum1/1
  Demux1/2 -> Sum/2
  abc to dq/1 -> Demux1/1
  Demux1/3 -> Terminator/1
  abc/1 -> abc to dq/1
  wt/1 -> abc to dq/2
  Vgq/1 -> Sum/1
  Gain2/1 -> Sum/3
  Gain/1 -> Sum1/2
  Sum1/1 -> Transfer Fcn/1
  Sum/1 -> Transfer Fcn1/1
  Transfer Fcn1/1 -> P/1, Gain/1

== system Hybrid_PV_Wind_System/January/RSC ==
  Vdc : Inport
  pwma : Inport  Port=2
  pwmb : Inport  Port=3
  pwmc : Inport  Port=4
  Fcn : Fcn  Expr=u(1)/6*(2*u(2)-u(3)-u(4))
  Fcn1 : Fcn  Expr=u(1)/6*(-u(2)+2*u(3)-u(4))
  Fcn2 : Fcn  Expr=u(1)/6*(-u(2)-u(3)+2*u(4))
  Mux : Mux
  Mux1 : Mux  Inputs=3
  Scope4 : Scope
  Via : Outport
  Vib : Outport  Port=2
  Vic : Outport  Port=3
  wires:
  Vdc/1 -> Mux/1
  Mux/1 -> Fcn2/1, Fcn1/1, Fcn/1
  pwma/1 -> Mux/2
  pwmb/1 -> Mux/3
  pwmc/1 -> Mux/4
  Fcn/1 -> Mux1/1, Via/1
  Fcn1/1 -> Vib/1, Mux1/2
  Fcn2/1 -> Vic/1, Mux1/3
  Mux1/1 -> Scope4/1

== system Hybrid_PV_Wind_System/January/T cell 1 ==
  T : Inport
  G : Inport  Port=2
  Add : Sum  Inputs=+-
  Add1 : Sum
  Constant2 : Constant  Value=NOCT
  Constant4 : Constant  Value=20
  Gain1 : Gain  Gain=1/80
  Gain2 : Gain  Gain=1/10
  Product3 : Product
  Tc : Outport
  wires:
  Constant2/1 -> Add/1
  Product3/1 -> Gain1/1
  Constant4/1 -> Add/2
  Add/1 -> Product3/1
  Gain2/1 -> Product3/2
  Gain1/1 -> Add1/1
  G/1 -> Gain2/1
  T/1 -> Add1/2
  Add1/1 -> Tc/1

== system Hybrid_PV_Wind_System/January/Temperature ==
  Demux : Demux  Tag=STV Demux  Outputs=1
      settings: DisplayOption=none
  FromWs : FromWorkspace  Tag=STV FromWs  VariableName=tuvar
      SigBuilderData=|
      | common.afterFinalStr = 'Extrapolate'
      | common.sampleTime = 0
      | dataSet.timeRange = [0 745]
      | dataSet.name = 'Group 1'
      | sbobj.Groups.Name = 'Group 1'
      | sbobj.Groups.Signals.Name = 'Signal 1'
      | sbobj.Groups.Signals.XData = [0 1 2 3 4 5 6 7 8 9 10 11 ... (745 elements, 1x745)]
      | sbobj.Groups.Signals.YData = [13.8 13.1 12.5 12.2 11.9 11.7 11.5 11.5 12.9 15.2 17.8 20.2 ... (745 elements, 1x745)]
      | sbobj.Groups.TimeRange = [0 745]
  Signal 1 : Outport  Tag=STV Outport
  wires:
  FromWs/1 -> Demux/1
  Demux/1 -> Signal 1/1

== system Hybrid_PV_Wind_System/January/Three Phase DC AC inverter ==
  Vdc : Inport
  pwma : Inport  Port=2
  pwmb : Inport  Port=3
  pwmc : Inport  Port=4
  Fcn : Fcn  Expr=u(1)/6*(2*u(2)-u(3)-u(4))
  Fcn1 : Fcn  Expr=u(1)/6*(-u(2)+2*u(3)-u(4))
  Fcn2 : Fcn  Expr=u(1)/6*(-u(2)-u(3)+2*u(4))
  Mux : Mux
  Via : Outport
  Vib : Outport  Port=2
  Vic : Outport  Port=3
  wires:
  Vdc/1 -> Mux/1
  Mux/1 -> Fcn2/1, Fcn1/1, Fcn/1
  Fcn2/1 -> Vic/1
  Fcn1/1 -> Vib/1
  Fcn/1 -> Via/1
  pwma/1 -> Mux/2
  pwmb/1 -> Mux/3
  pwmc/1 -> Mux/4

== system Hybrid_PV_Wind_System/January/Turbine1 ==
  note: T_aero
  note: omega_t
  note: omega
  note: lambda
  note: Cp
  S : Inport
  B : Inport  Port=2
  1/lambda_i : Fcn  Expr=1/(u(1)+0.08*u(2))-0.035/(2^3+1)
  Cp(lambda,B) : Fcn  Expr=0.5176*(116*u(2)-0.4*u(3)-5)*exp(-21*u(2))+0.0068*u(1)
  Gain : Gain  Gain=R_/G
  Gain1 : Gain  Gain=1/G
  Gain2 : Gain  Gain=1/G
  Gain3 : Gain  Gain=lambda_opt*G/R_
  Gain5 : Gain  Gain=-1
  Mux : Mux  Inputs=2
  Mux1 : Mux  Inputs=3
  Mux2 : Mux  Inputs=3
  Mux3 : Mux  Inputs=2
  Product : Product  Inputs=*/
  Saturation : Saturate  UpperLimit=200  LowerLimit=0
  Saturation1 : Saturate  UpperLimit=0  LowerLimit=-3e6
  Saturation2 : Saturate  UpperLimit=200  LowerLimit=0
  Scope{1..5} (5 alike) : Scope
  Subsystem : Subsystem
  Subsystem1 : Subsystem
  Subsystem8 : Subsystem
  Taero(S,cp) : Fcn  Expr=0.5*u(1)*Rho*pi*(R_^2)*(u(2)^3)/u(3)
  omega : Outport
  Ps* : Outport  Port=2
  wires:
  Subsystem8/1(Ps*) -> Saturation1/1
  1/lambda_i/1 -> Mux1/2
  B/1 -> Mux1/3, Mux3/2
  Product/1 -> Mux3/1, Mux1/1
  S/1 -> Gain3/1, Mux2/2, Product/2
  Cp(lambda,B)/1 -> Mux2/1
  Gain/1 -> Product/1
  Gain2/1 -> Mux2/3
  Mux1/1 -> Cp(lambda,B)/1
  Mux2/1 -> Taero(S,cp)/1
  Taero(S,cp)/1 -> Gain1/1
  Mux/1 -> Scope1/1
  Mux3/1 -> 1/lambda_i/1
  Gain5/1 -> Subsystem8/1(Tem*), Scope3/1
  Subsystem1/1(Tem) -> Subsystem/2(Tem), Gain5/1
  Gain1/1 -> Scope5/1, Subsystem1/1(Tt), Subsystem/1(Tt)
  Gain3/1 -> Saturation/1, Mux/1
  Saturation/1 -> Subsystem1/2(omega_ref)
  Saturation1/1 -> Scope4/1, Ps*/1
  Subsystem/1(omega) -> Saturation2/1
  Saturation2/1 -> omega/1, Scope2/1, Gain/1, Gain2/1, Mux/2, Subsystem1/3(omega), Subsystem8/2(omega)

== system Hybrid_PV_Wind_System/January/Wind speed ==
  Demux : Demux  Tag=STV Demux  Outputs=1
      settings: DisplayOption=none
  FromWs : FromWorkspace  Tag=STV FromWs  VariableName=tuvar
      SigBuilderData=|
      | common.afterFinalStr = 'Extrapolate'
      | common.sampleTime = 0
      | dataSet.timeRange = [0 750]
      | dataSet.name = 'Group 1'
      | sbobj.Groups.Name = 'Group 1'
      | sbobj.Groups.Signals.Name = 'Signal 2'
      | sbobj.Groups.Signals.XData = [0 1 2 3 4 5 6 7 8 9 10 11 ... (745 elements, 1x745)]
      | sbobj.Groups.Signals.YData = [3 2.6 2.7 3 2.5 2.7 2.3 3 2.9 4.9 4.6 4.9 ... (745 elements, 1x745)]
      | sbobj.Groups.TimeRange = [0 750]
  Signal 2 : Outport  Tag=STV Outport
  wires:
  FromWs/1 -> Demux/1
  Demux/1 -> Signal 2/1

== system Hybrid_PV_Wind_System/January/control PWW  ==
  note: PI
  note: Iq*
  note: Vq*
  note: Vd*
  note: Id*
  note: Vdc*
  note: PI
  note: PI
  Id : Inport
  Iq : Inport  Port=2
  Vdc : Inport  Port=3
  wt : Inport  Port=4
  Irq : Inport  Port=5
  Vgq : Inport  Port=6
  Constant : Constant  Value=0
  Constant2 : Constant  Value=Id_
  Constant3 : Constant  Value=0
  Constant4 : Constant  Value=Vdc_
  Gain : Gain  Gain=L*Ws
  Gain1 : Gain  Gain=L*Ws
  Mux1 : Mux  Inputs=2
  Mux2 : Mux  Inputs=3
  Mux3 : Mux  Inputs=2
  Mux4 : Mux  Inputs=2
  PI : Subsystem
  PI1 : Subsystem
  PI2 : Subsystem
  Scope{1..3,5} (4 alike) : Scope
  Sum{,1..2,5} (4 alike) : Sum  Inputs=|+-
  Sum4 : Sum  Inputs=+++
  Sum6 : Sum  Inputs=++-
  dq0 to abc1 : powerlib_meascontrol/Transformations/dq0 to abc  Alignment=90 degrees behind phase A axis
  abc_ref : Outport
  wires:
  Sum1/1 -> PI1/1(e)
  Sum/1 -> PI/1(e)
  PI/1(s) -> Sum2/1
  Constant2/1 -> Mux1/1, Sum1/1
  PI1/1(s) -> Sum4/2
  Constant3/1 -> Mux2/3
  Mux2/1 -> dq0 to abc1/1, Scope5/1
  dq0 to abc1/1 -> abc_ref/1
  wt/1 -> dq0 to abc1/2
  PI2/1(s) -> Sum6/2
  Id/1 -> Mux1/2, Sum1/2, Gain/1
  Sum6/1 -> Mux2/2
  Sum5/1 -> PI2/1(e)
  Sum4/1 -> Mux2/1
  Vgq/1 -> Sum6/1
  Gain/1 -> Sum6/3
  Irq/1 -> Sum2/2
  Constant/1 -> Sum4/1
  Gain1/1 -> Sum4/3
  Mux1/1 -> Scope1/1
  Sum2/1 -> Sum5/1, Mux3/1
  Iq/1 -> Sum5/2, Mux3/2, Gain1/1
  Mux3/1 -> Scope2/1
  Constant4/1 -> Mux4/1, Sum/1
  Vdc/1 -> Mux4/2, Sum/2
  Mux4/1 -> Scope3/1

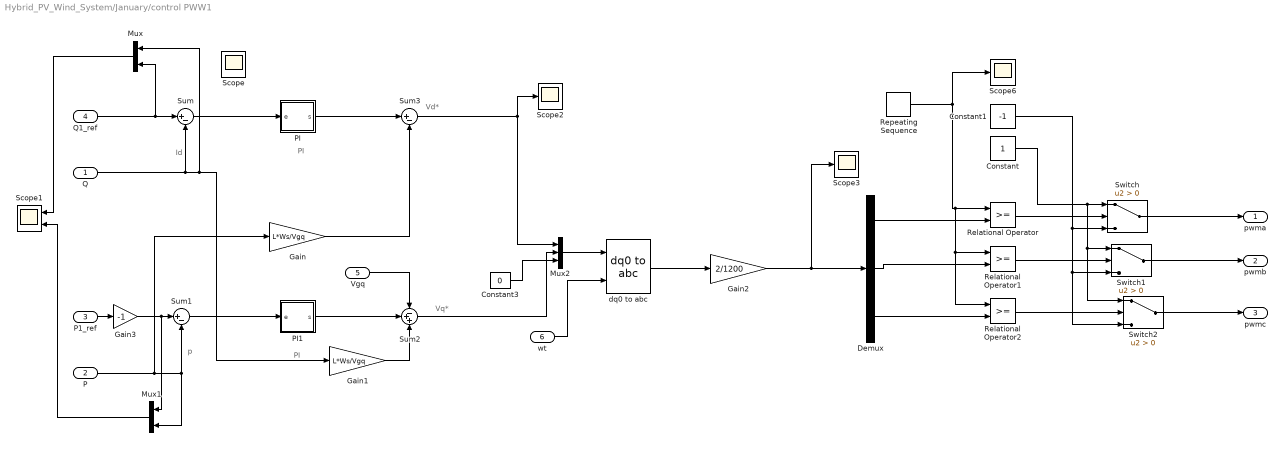
== system Hybrid_PV_Wind_System/January/control PWW1 ==
  note: PI
  note: PI
  note: Vd*
  note: Vq*
  note: p
  note: Id
  "Q " : Inport
  P : Inport  Port=2
  P1_ref : Inport  Port=3
  Q1_ref : Inport  Port=4
  Vgq : Inport  Port=5
  wt : Inport  Port=6
  Constant : Constant
  Constant1 : Constant  Value=-1
  Constant3 : Constant  Value=0
  Demux : Demux  Outputs=3
  Gain : Gain  Gain=L*Ws/Vgq
  Gain1 : Gain  Gain=L*Ws/Vgq
  Gain2 : Gain  Gain=2/1200
  Gain3 : Gain  Gain=-1
  Mux : Mux  Inputs=2
  Mux1 : Mux  Inputs=2
  Mux2 : Mux  Inputs=3
  PI : Subsystem
  PI1 : Subsystem
  Relational Operator : RelationalOperator  OutDataTypeStr=boolean  RndMeth=Nearest
  Relational Operator1 : RelationalOperator  OutDataTypeStr=boolean  RndMeth=Nearest
  Relational Operator2 : RelationalOperator  OutDataTypeStr=boolean  RndMeth=Nearest
  Repeating Sequence : simulink/Sources/Repeating Sequence  rep_seq_t=[0 1/40000 1/20000 3/40000 1/10000]  rep_seq_y="[0 1  0 -1 0]"
  Scope{,2..3,6} (4 alike) : Scope
  Scope1 : Scope  NumInputPorts=2
  Sum : Sum  Inputs=|+-
  Sum1 : Sum  Inputs=|+-
  Sum2 : Sum  Inputs=-++
  Sum3 : Sum  Inputs=|+-
  Switch : Switch  Criteria=u2 > Threshold
  Switch1 : Switch  Criteria=u2 > Threshold
  Switch2 : Switch  Criteria=u2 > Threshold
  dq0 to abc : powerlib_meascontrol/Transformations/dq0 to abc  Alignment=90 degrees behind phase A axis
  pwma : Outport
  pwmb : Outport  Port=2
  pwmc : Outport  Port=3
  wires:
  Sum1/1 -> PI1/1(e)
  "Q "/1 -> Mux/1, Gain1/1, Sum/2
  Sum/1 -> PI/1(e)
  PI/1(s) -> Sum3/1
  P1_ref/1 -> Gain3/1
  Mux/1 -> Scope1/1
  P/1 -> Mux1/2, Sum1/2, Gain/1
  Mux1/1 -> Scope1/2
  PI1/1(s) -> Sum2/2
  Constant3/1 -> Mux2/3
  Q1_ref/1 -> Mux/2, Sum/1
  Repeating Sequence/1 -> Scope6/1, Relational Operator2/1, Relational Operator1/1, Relational Operator/1
  Demux/1 -> Relational Operator/2
  Demux/2 -> Relational Operator1/2
  Demux/3 -> Relational Operator2/2
  Switch2/1 -> pwmc/1
  Switch1/1 -> pwmb/1
  Switch/1 -> pwma/1
  Relational Operator/1 -> Switch/2
  Constant/1 -> Switch1/1, Switch2/1, Switch/1
  Constant1/1 -> Switch/3, Switch1/3, Switch2/3
  Relational Operator1/1 -> Switch1/2
  Relational Operator2/1 -> Switch2/2
  Mux2/1 -> dq0 to abc/1
  Sum3/1 -> Scope2/1, Mux2/1
  Sum2/1 -> Mux2/2
  wt/1 -> dq0 to abc/2
  Vgq/1 -> Sum2/1
  Gain/1 -> Sum3/2
  Gain1/1 -> Sum2/3
  dq0 to abc/1 -> Gain2/1
  Gain2/1 -> Scope3/1, Demux/1
  Gain3/1 -> Mux1/1, Sum1/1

== system Hybrid_PV_Wind_System/August/Turbine/Subsystem ==
  Tt : Inport
  Tem : Inport  Port=2
  Add : Sum  Inputs=+--
  Gain6 : Gain  Gain=1/J
  Gain7 : Gain  Gain=f
  Integrator : Integrator  InitialCondition=64.5  LowerSaturationLimit=1e-5
  omega : Outport
  wires:
  Add/1 -> Gain6/1
  Integrator/1 -> omega/1, Gain7/1
  Gain6/1 -> Integrator/1
  Tt/1 -> Add/1
  Gain7/1 -> Add/3
  Tem/1 -> Add/2

== system Hybrid_PV_Wind_System/August/Turbine/Subsystem1 ==
  Tt : Inport
  omega_ref : Inport  Port=2
  omega : Inport  Port=3
  Add : Sum  Inputs=+-
  PID Controller : simulink/Continuous/PID Controller  Controller=PI  Form=Parallel  TimeDomain=Continuous-time  SampleTime=-1  IntegratorMethod=Forward Euler  ControllerParametersSource=internal  P=J  I=f  D=0  N=100  UseFilter=on  TunerSelectOption=Transfer Function Based (PID Tuner App)  InitialConditionSource=internal  InitialConditionForIntegrator=0  InitialConditionForFilter=0  DifferentiatorICPrevScaledInput=0  ExternalReset=none  TrackingMode=off  Kt=1  LimitOutput=off  UpperSaturationLimit=inf  LowerSaturationLimit=0  LinearizeAsGain=on  AntiWindupMode=none  Kb=1  POutMin=[]  POutMax=[]  IOutMin=[]  IOutMax=[]  DOutMin=[]  DOutMax=[]  NOutMin=[]  NOutMax=[]  SumOutMin=[]  SumOutMax=[]  SaturationOutMin=[]  SaturationOutMax=[]  PParamMin=[]  PParamMax=[]  IParamMin=[]  IParamMax=[]  DParamMin=[]  DParamMax=[]  NParamMin=[]  NParamMax=[]  KbParamMin=[]  KbParamMax=[]  KtParamMin=[]  KtParamMax=[]  KbOutMin=[]  KbOutMax=[]  KtOutMin=[]  KtOutMax=[]  IntegratorOutMin=[]  IntegratorOutMax=[]  FilterOutMin=[]  FilterOutMax=[]  SumI1OutMin=[]  SumI1OutMax=[]  SumI2OutMin=[]  SumI2OutMax=[]  SumI3OutMin=[]  SumI3OutMax=[]  SumDOutMin=[]  SumDOutMax=[]  DifferentiatorOutMin=[]  DifferentiatorOutMax=[]  FilterDiffOutCoefMin=[]  FilterDiffOutCoefMax=[]  ReciprocalOutMin=[]  ReciprocalOutMax=[]  SumDenOutMin=[]  SumDenOutMax=[]  SumNumOutMin=[]  SumNumOutMax=[]  DivideOutMin=[]  DivideOutMax=[]  IntegratorContinuousStateAttributes=''  IntegratorStateMustResolveToSignalObject=off  IntegratorRTWStateStorageClass=Auto  FilterContinuousStateAttributes=''  FilterStateMustResolveToSignalObject=off  FilterRTWStateStorageClass=Auto
  Saturation : Saturate  UpperLimit=1.9e4  LowerLimit=0
  Sum3 : Sum  Inputs=|+-
  Tem : Outport
  wires:
  Tt/1 -> Add/1
  Saturation/1 -> Tem/1
  Add/1 -> Saturation/1
  PID Controller/1 -> Add/2
  omega_ref/1 -> Sum3/1
  Sum3/1 -> PID Controller/1
  omega/1 -> Sum3/2

== system Hybrid_PV_Wind_System/August/Turbine/Subsystem8 ==
  Tem* : Inport
  omega : Inport  Port=2
  Gain : Gain
  Mux : Mux  Inputs=2
  fcn2 : Fcn  Expr=u(1)*u(2)
  Ps* : Outport
  wires:
  Gain/1 -> Mux/2
  Tem*/1 -> Mux/1
  fcn2/1 -> Ps*/1
  omega/1 -> Gain/1
  Mux/1 -> fcn2/1

== system Hybrid_PV_Wind_System/August/control PWW /PI ==
  e : Inport
  Add : Sum
  Gain : Gain  Gain=1.45
  Gain1 : Gain  Gain=27.27
  Integrator : Integrator  UpperSaturationLimit=350  LowerSaturationLimit=-350
  s : Outport
  wires:
  Gain/1 -> Add/1
  Gain1/1 -> Integrator/1
  Integrator/1 -> Add/2
  e/1 -> Gain/1, Gain1/1
  Add/1 -> s/1

== system Hybrid_PV_Wind_System/August/control PWW /PI1 ==
  e : Inport
  Add : Sum
  Gain : Gain  Gain=kp
  Gain1 : Gain  Gain=ki
  Integrator : Integrator  UpperSaturationLimit=600  LowerSaturationLimit=-600
  s : Outport
  wires:
  Add/1 -> s/1
  e/1 -> Gain/1, Gain1/1
  Integrator/1 -> Add/2
  Gain1/1 -> Integrator/1
  Gain/1 -> Add/1

== system Hybrid_PV_Wind_System/August/control PWW /PI2 ==
  e : Inport
  Add : Sum
  Gain : Gain  Gain=kp
  Gain1 : Gain  Gain=ki
  Integrator : Integrator  UpperSaturationLimit=600  LowerSaturationLimit=-600
  s : Outport
  wires:
  Add/1 -> s/1
  e/1 -> Gain/1, Gain1/1
  Integrator/1 -> Add/2
  Gain1/1 -> Integrator/1
  Gain/1 -> Add/1

== system Hybrid_PV_Wind_System/August/control PWW1/PI ==
  e : Inport
  Add : Sum  Inputs=--
  Gain : Gain  Gain=kp1
  Gain1 : Gain  Gain=ki1
  Integrator : Integrator  UpperSaturationLimit=350  LowerSaturationLimit=-350
  s : Outport
  wires:
  Gain/1 -> Add/1
  Gain1/1 -> Integrator/1
  Integrator/1 -> Add/2
  e/1 -> Gain/1, Gain1/1
  Add/1 -> s/1

== system Hybrid_PV_Wind_System/August/control PWW1/PI1 ==
  e : Inport
  Add : Sum  Inputs=--
  Gain : Gain  Gain=kp
  Gain1 : Gain  Gain=ki
  Integrator : Integrator  UpperSaturationLimit=350  LowerSaturationLimit=-350
  s : Outport
  wires:
  Add/1 -> s/1
  e/1 -> Gain/1, Gain1/1
  Integrator/1 -> Add/2
  Gain1/1 -> Integrator/1
  Gain/1 -> Add/1

== system Hybrid_PV_Wind_System/January/Turbine1/Subsystem ==
  Tt : Inport
  Tem : Inport  Port=2
  Add : Sum  Inputs=+--
  Gain6 : Gain  Gain=1/J
  Gain7 : Gain  Gain=f
  Integrator : Integrator  InitialCondition=64.5  LowerSaturationLimit=1e-5
  omega : Outport
  wires:
  Add/1 -> Gain6/1
  Integrator/1 -> omega/1, Gain7/1
  Gain6/1 -> Integrator/1
  Tt/1 -> Add/1
  Gain7/1 -> Add/3
  Tem/1 -> Add/2

== system Hybrid_PV_Wind_System/January/Turbine1/Subsystem1 ==
  Tt : Inport
  omega_ref : Inport  Port=2
  omega : Inport  Port=3
  Add : Sum  Inputs=+-
  PID Controller : simulink/Continuous/PID Controller  Controller=PI  Form=Parallel  TimeDomain=Continuous-time  SampleTime=-1  IntegratorMethod=Forward Euler  ControllerParametersSource=internal  P=J  I=f  D=0  N=100  UseFilter=on  TunerSelectOption=Transfer Function Based (PID Tuner App)  InitialConditionSource=internal  InitialConditionForIntegrator=0  InitialConditionForFilter=0  DifferentiatorICPrevScaledInput=0  ExternalReset=none  TrackingMode=off  Kt=1  LimitOutput=off  UpperSaturationLimit=inf  LowerSaturationLimit=0  LinearizeAsGain=on  AntiWindupMode=none  Kb=1  POutMin=[]  POutMax=[]  IOutMin=[]  IOutMax=[]  DOutMin=[]  DOutMax=[]  NOutMin=[]  NOutMax=[]  SumOutMin=[]  SumOutMax=[]  SaturationOutMin=[]  SaturationOutMax=[]  PParamMin=[]  PParamMax=[]  IParamMin=[]  IParamMax=[]  DParamMin=[]  DParamMax=[]  NParamMin=[]  NParamMax=[]  KbParamMin=[]  KbParamMax=[]  KtParamMin=[]  KtParamMax=[]  KbOutMin=[]  KbOutMax=[]  KtOutMin=[]  KtOutMax=[]  IntegratorOutMin=[]  IntegratorOutMax=[]  FilterOutMin=[]  FilterOutMax=[]  SumI1OutMin=[]  SumI1OutMax=[]  SumI2OutMin=[]  SumI2OutMax=[]  SumI3OutMin=[]  SumI3OutMax=[]  SumDOutMin=[]  SumDOutMax=[]  DifferentiatorOutMin=[]  DifferentiatorOutMax=[]  FilterDiffOutCoefMin=[]  FilterDiffOutCoefMax=[]  ReciprocalOutMin=[]  ReciprocalOutMax=[]  SumDenOutMin=[]  SumDenOutMax=[]  SumNumOutMin=[]  SumNumOutMax=[]  DivideOutMin=[]  DivideOutMax=[]  IntegratorContinuousStateAttributes=''  IntegratorStateMustResolveToSignalObject=off  IntegratorRTWStateStorageClass=Auto  FilterContinuousStateAttributes=''  FilterStateMustResolveToSignalObject=off  FilterRTWStateStorageClass=Auto
  Saturation : Saturate  UpperLimit=1.9e4  LowerLimit=0
  Sum3 : Sum  Inputs=|+-
  Tem : Outport
  wires:
  Tt/1 -> Add/1
  Saturation/1 -> Tem/1
  Add/1 -> Saturation/1
  PID Controller/1 -> Add/2
  omega_ref/1 -> Sum3/1
  Sum3/1 -> PID Controller/1
  omega/1 -> Sum3/2

== system Hybrid_PV_Wind_System/January/Turbine1/Subsystem8 ==
  Tem* : Inport
  omega : Inport  Port=2
  Gain : Gain
  Mux : Mux  Inputs=2
  fcn2 : Fcn  Expr=u(1)*u(2)
  Ps* : Outport
  wires:
  Gain/1 -> Mux/2
  Tem*/1 -> Mux/1
  fcn2/1 -> Ps*/1
  omega/1 -> Gain/1
  Mux/1 -> fcn2/1

== system Hybrid_PV_Wind_System/January/control PWW /PI ==
  e : Inport
  Add : Sum
  Gain : Gain  Gain=1.45
  Gain1 : Gain  Gain=27.27
  Integrator : Integrator  UpperSaturationLimit=350  LowerSaturationLimit=-350
  s : Outport
  wires:
  Gain/1 -> Add/1
  Gain1/1 -> Integrator/1
  Integrator/1 -> Add/2
  e/1 -> Gain/1, Gain1/1
  Add/1 -> s/1

== system Hybrid_PV_Wind_System/January/control PWW /PI1 ==
  e : Inport
  Add : Sum
  Gain : Gain  Gain=kp
  Gain1 : Gain  Gain=ki
  Integrator : Integrator  UpperSaturationLimit=600  LowerSaturationLimit=-600
  s : Outport
  wires:
  Add/1 -> s/1
  e/1 -> Gain/1, Gain1/1
  Integrator/1 -> Add/2
  Gain1/1 -> Integrator/1
  Gain/1 -> Add/1

== system Hybrid_PV_Wind_System/January/control PWW /PI2 ==
  e : Inport
  Add : Sum
  Gain : Gain  Gain=kp
  Gain1 : Gain  Gain=ki
  Integrator : Integrator  UpperSaturationLimit=600  LowerSaturationLimit=-600
  s : Outport
  wires:
  Add/1 -> s/1
  e/1 -> Gain/1, Gain1/1
  Integrator/1 -> Add/2
  Gain1/1 -> Integrator/1
  Gain/1 -> Add/1

== system Hybrid_PV_Wind_System/January/control PWW1/PI ==
  e : Inport
  Add : Sum  Inputs=--
  Gain : Gain  Gain=kp1
  Gain1 : Gain  Gain=ki1
  Integrator : Integrator  UpperSaturationLimit=350  LowerSaturationLimit=-350
  s : Outport
  wires:
  Gain/1 -> Add/1
  Gain1/1 -> Integrator/1
  Integrator/1 -> Add/2
  e/1 -> Gain/1, Gain1/1
  Add/1 -> s/1

== system Hybrid_PV_Wind_System/January/control PWW1/PI1 ==
  e : Inport
  Add : Sum  Inputs=--
  Gain : Gain  Gain=kp
  Gain1 : Gain  Gain=ki
  Integrator : Integrator  UpperSaturationLimit=350  LowerSaturationLimit=-350
  s : Outport
  wires:
  Add/1 -> s/1
  e/1 -> Gain/1, Gain1/1
  Integrator/1 -> Add/2
  Gain1/1 -> Integrator/1
  Gain/1 -> Add/1

== matlab function Hybrid_PV_Wind_System/January/Gm1/Irradiation ==
  data: i input; k input; y output; o input; p input
function y= fcn(i,k,o,p)
%Solar irradiation
%k=DNI   o=DHI    p=GHI
n=0;
phi=27.87429;            %latitude
L_st=0;           %standard meridian 
L_loc=-0.29388;          %longitude
c=0;              %daylight savings
theta_m=23;        %tilt angle
phi_m=180;          %solar module azimuth
rho=0.2;            %ground albedo
T_off=1;          %time difference

SVF=0.5*(1+cosd(theta_m));
G_gnd=p*rho*(1-SVF);


 
  n=ceil(i/24);
  C=0.095+0.04*sind(360*(n-100)/365);
  delta=23.45*sind(360*(n-80)/365);  
  B=(n-1)*360/365;
  ET=229.2*(0.000075+0.001868*cosd(B)-0.032077*sind(B)-0.014615*cosd(2*B)-0.04089*sind(2*B));
  %cos(w_)=-tan(phi)+tan(delta);
  G_dif=C*p*SVF;
  
  
      
      UT=(i/24-fix(i/24))*24-T_off;
      t=UT+ET+4;%*(L_st-L_loc)+c;
    
      w=15*(UT-12);
      D=sind(delta)*sind(phi)+cosd(delta)*cosd(phi)*cosd(w);              %sin(a)
      
      %E=sin(phi)*sin(delta)+cos(phi)*cos(delta)*cos(w);             %cos(theta_z)
      %z=x*E+y;                                                      %GHI
      A=(cosd(phi)*sind(delta)-cosd(delta)*sind(phi)*cosd(w))/cosd(asind(D));     %cos(phi_s')
      
      
if w>0
    
    phi_s=360-acosd(complex(A));
    
else
    
    phi_s=acosd(complex(A));
    
end

      F=cosd(asind(complex(D)))*cosd(phi_s-phi_m)*sind(theta_m)+D*cosd(theta_m);    %cos(gama)
    
          G_dir=k*F;
   
          
      G=G_dir+G_dif+G_gnd;
    
y = real(G);

== matlab function Hybrid_PV_Wind_System/August/Gm1/Irradiation ==
  data: i input; k input; y output; o input; p input
function y= fcn(i,k,o,p)
%Solar irradiation
%k=DNI   o=DHI    p=GHI
n=0;
phi=27.87429;            %latitude
L_st=0;           %standard meridian 
L_loc=-0.29388;          %longitude
c=0;              %daylight savings
theta_m=23;        %tilt angle
phi_m=180;          %solar module azimuth
rho=0.2;            %ground albedo
T_off=1;          %time difference

SVF=0.5*(1+cosd(theta_m));
G_gnd=p*rho*(1-SVF);


 
  n=ceil(i/24);
  C=0.095+0.04*sind(360*(n-100)/365);
  delta=23.45*sind(360*(n-80)/365);  
  B=(n-1)*360/365;
  ET=229.2*(0.000075+0.001868*cosd(B)-0.032077*sind(B)-0.014615*cosd(2*B)-0.04089*sind(2*B));
  %cos(w_)=-tan(phi)+tan(delta);
  G_dif=C*p*SVF;
  
  
      
      UT=(i/24-fix(i/24))*24-T_off;
      t=UT+ET+4;%*(L_st-L_loc)+c;
    
      w=15*(UT-12);
      D=sind(delta)*sind(phi)+cosd(delta)*cosd(phi)*cosd(w);              %sin(a)
      
      %E=sin(phi)*sin(delta)+cos(phi)*cos(delta)*cos(w);             %cos(theta_z)
      %z=x*E+y;                                                      %GHI
      A=(cosd(phi)*sind(delta)-cosd(delta)*sind(phi)*cosd(w))/cosd(asind(D));     %cos(phi_s')
      
      
if w>0
    
    phi_s=360-acosd(complex(A));
    
else
    
    phi_s=acosd(complex(A));
    
end

      F=cosd(asind(complex(D)))*cosd(phi_s-phi_m)*sind(theta_m)+D*cosd(theta_m);    %cos(gama)
    
          G_dir=k*F;
   
          
      G=G_dir+G_dif+G_gnd;
    
y = real(G);

== matlab function Hybrid_PV_Wind_System/August/MPPT1/CI ==
  data: DV input; DP input; d output
function d=PO(DV,DP)
persistent   v ;

if isempty(v)
    v=37.9;
end

if(DP==0)
else
    if(DP>0)
        if(DV>0)
                v=v+0.01;
            else
                v=v-0.01;
           end 
       else
        if(DV>0)
                v=v-0.01;
            else
                v=v+0.01;
        end
    end
end

d=v;
end

== matlab function Hybrid_PV_Wind_System/January/MPPT1/CI ==
  data: DV input; DP input; d output
function d=PO(DV,DP)
persistent   v ;

if isempty(v)
    v=37.9;
end

if(DP==0)
else
    if(DP>0)
        if(DV>0)
                v=v+0.01;
            else
                v=v-0.01;
           end 
       else
        if(DV>0)
                v=v-0.01;
            else
                v=v+0.01;
        end
    end
end

d=v;
end
